simulink model "test_ones"  (R2017b)
settings: Solver=FixedStepDiscrete  StartTime=0.0  StopTime=10.0  FixedStep=0.100000  RelTol=1e-3
model workspace (MAT data in the model file):
  already_pp = 1
settings Model: Creator=fconzelm  LastModifiedBy=hbourbou
settings DebuggingCC: AlgebraicLoopMsg=error  ArtificialAlgebraicLoopMsg=error  SingleTaskRateTransMsg=error

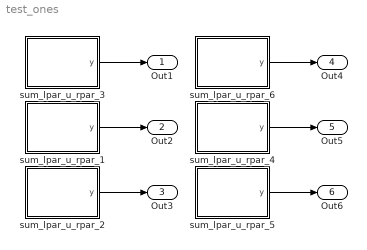
== system test_ones ==
  sum_lpar_u_rpar_1 : MATLAB Function  TreatAsAtomicUnit=on
  sum_lpar_u_rpar_2 : MATLAB Function  TreatAsAtomicUnit=on
  sum_lpar_u_rpar_3 : MATLAB Function  TreatAsAtomicUnit=on
  sum_lpar_u_rpar_4 : MATLAB Function  TreatAsAtomicUnit=on
  sum_lpar_u_rpar_5 : MATLAB Function  TreatAsAtomicUnit=on
  sum_lpar_u_rpar_6 : MATLAB Function  TreatAsAtomicUnit=on
  Out1 : Outport
  Out2 : Outport  Port=2
  Out3 : Outport  Port=3
  Out4 : Outport  Port=4
  Out5 : Outport  Port=5
  Out6 : Outport  Port=6
  wires:
  sum_lpar_u_rpar_3/1(y) -> Out1/1
  sum_lpar_u_rpar_1/1(y) -> Out2/1
  sum_lpar_u_rpar_2/1(y) -> Out3/1
  sum_lpar_u_rpar_6/1(y) -> Out4/1
  sum_lpar_u_rpar_4/1(y) -> Out5/1
  sum_lpar_u_rpar_5/1(y) -> Out6/1

== matlab function test_ones/sum_lpar_u_rpar_1 ==
  data: y output
function y = ones1()

y = ones([1, 3]);

== matlab function test_ones/sum_lpar_u_rpar_2 ==
  data: y output
function y = ones1()

y = ones([1, 2, 3]);

== matlab function test_ones/sum_lpar_u_rpar_3 ==
  data: y output
function y = ones1()

y = ones(1);

== matlab function test_ones/sum_lpar_u_rpar_4 ==
  data: y output
function y = ones1()

y = ones(1, 3);

== matlab function test_ones/sum_lpar_u_rpar_5 ==
  data: y output
function y = ones1()

y = ones(1, 2, 3);

== matlab function test_ones/sum_lpar_u_rpar_6 ==
  data: y output
function y = ones1()

y = ones(1, 1);
